simulink model "proj1"  (Simulink 7.7)
settings: Solver=ode45  StartTime=0.0  StopTime=30  RelTol=1e-3
values from neighbouring files (symbols this model uses):
  B = -inv(A)*C    [proj.m]
  Cir = fill(x1,y1,'r')    [proj.m]
  D = -inv(A)*G    [proj.m]
  K = lqr(T,Q,Qr,R)    [proj.m]
  Q = [0;0;Q]    [proj.m]
  Squ = fill(x2,y2,'b')    [proj.m]
undefined symbols (not defined in the file or in its folder): sigbuilder_block, simule
settings Model: Creator=Owner  LastModifiedBy=Owner
settings OptimizationCC: InlineInvariantSignals=on  InitFltsAndDblsToZero=on
settings DebuggingCC: SaveWithParameterizedLinksMsg=none  SignalResolutionControl=TryResolveAllWithWarning  MultiTaskDSMMsg=warning  MultiTaskCondExecSysMsg=none  StrictBusMsg=None
settings RTWCC: IncludeERTFirstTime=on
settings GRTTargetCC: TargetFcnLib=ansi_tfl_tmw.mat

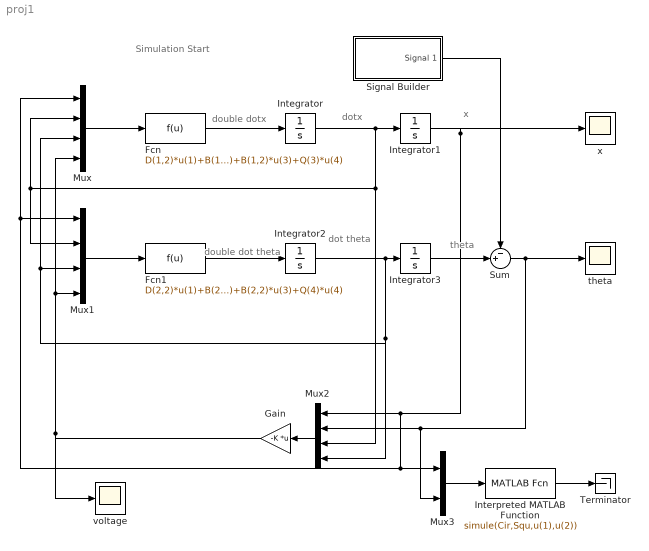
== system proj1 ==
  note: x
  note: dotx
  note: double dotx
  note: double dot
      | theta
  note: dot theta
  note: theta
  note: Simulation Start
  Fcn : Fcn  Expr=D(1,2)*u(1)+B(1,1)*u(2)+B(1,2)*u(3)+Q(3)*u(4)
  Fcn1 : Fcn  Expr=D(2,2)*u(1)+B(2,1)*u(2)+B(2,2)*u(3)+Q(4)*u(4)
  Gain : Gain  Gain=-K  Multiplication=Matrix(K*u)
  Integrator : Integrator
  Integrator1 : Integrator
  Integrator2 : Integrator
  Integrator3 : Integrator  InitialCondition=0.5
  Interpreted MATLAB Function : MATLABFcn  MATLABFcn=simule(Cir,Squ,u(1),u(2))
  Mux : Mux
  Mux1 : Mux
  Mux2 : Mux
  Mux3 : Mux  Inputs=2
  Signal Builder : Subsystem  Tag=STV Subsys  LoadFcn=sigbuilder_block('load');  StartFcn=sigbuilder_block('start');  StopFcn=sigbuilder_block('stop');  ClipboardFcn=sigbuilder_block('clipboard');  mask(Sigbuilder block){}
      mask help: Create and generate interchangeable groups of signals whose waveforms are piecewise linear.
      mask init:
      | if ~strcmp(get_param(bdroot(gcbh),'SimulationStatus'),'stopped') tuvar = sigbuilder_block('maskInit'); end
      settings: CopyFcn=sigbuilder_block('copy');  DeleteFcn=sigbuilder_block('delete');  ModelCloseFcn=sigbuilder_block('modelClose');  PreSaveFcn=sigbuilder_block('preSave');  NameChangeFcn=sigbuilder_block('namechange');  OpenFcn=sigbuilder_block('open',[107.25 99.75 550.5 399.75 ]);  CloseFcn=sigbuilder_block('close');
      mask Display: plot(0, 0, 100, 100,[2, 2, 32, 32, 2], [68, 8, 8, 68, 68],[32, 2], [38, 38], [32, 19, 2],[53, 60, 44], [32, 17, 17, 2],[16, 16, 31, 31]);txt = getActiveGroup(gcbh);text(2, 100, txt,'verticalAlignment', 'top');
  Sum : Sum  Inputs=-+|
  Terminator : Terminator
  theta : Scope
  voltage : Scope
      settings: YMin=-0.045  YMax=0.035  SaveName=ScopeData2
  x : Scope
  wires:
  Integrator/1 -> Mux/2, Mux1/2, Mux2/3, Integrator1/1
  Integrator1/1 -> Mux2/1, Mux3/1, Mux1/1, Mux/1, x/1
  Fcn/1 -> Integrator/1
  Mux/1 -> Fcn/1
  Integrator2/1 -> Integrator3/1, Mux1/3, Mux/3, Mux2/4
  Integrator3/1 -> Sum/2
  Fcn1/1 -> Integrator2/1
  Mux1/1 -> Fcn1/1
  Mux2/1 -> Gain/1
  Mux3/1 -> Interpreted MATLAB Function/1
  Interpreted MATLAB Function/1 -> Terminator/1
  Gain/1 -> Mux1/4, Mux/4, voltage/1
  Signal Builder/1(Signal 1) -> Sum/1
  Sum/1 -> theta/1, Mux2/2, Mux3/2

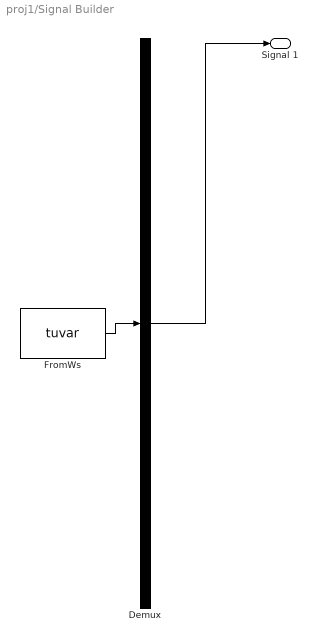
== system proj1/Signal Builder ==
  Demux : Demux  Tag=STV Demux  Outputs=1
  FromWs : FromWorkspace  Tag=STV FromWs  VariableName=tuvar  SampleTime=0  SigBuilderData=DataTag0  VnvData=DataTag1
      SigBuilderData=|
      | common.afterFinalStr = 'Extrapolate'
      | common.sampleTime = 0
      | dataSet.timeRange = [0 30]
      | dataSet.name = 'Group 1'
      | sbobj.Groups.Name = 'Group 1'
      | sbobj.Groups.Signals.Name = 'Signal 1'
      | sbobj.Groups.Signals.XData = [0 3.64 4 5.36 5.7 5.92 6.14 6.14 7.76 7.76 8.02 30]
      | sbobj.Groups.Signals.YData = [0 0 0.14 0.14 0.005 0.005 -0.002 0 0 -0.002 -0.002 0]
      | sbobj.Groups.TimeRange = [0 30]
  Signal 1 : Outport  Tag=STV Outport
  wires:
  Demux/1 -> Signal 1/1
  FromWs/1 -> Demux/1
